simulink model "frequency_syn"  (R2016a)
settings: Solver=VariableStepAuto  StartTime=0.0  StopTime=10.0  RelTol=1e-3
undefined symbols (not defined in the file or in its folder): j
libraries: dspobslib x3, commchan3 x2, commdigbbndpm3 x1, commrandsrc2 x1, dspxfrm3 x1
settings Model: Creator=dell  LastModifiedBy=dell

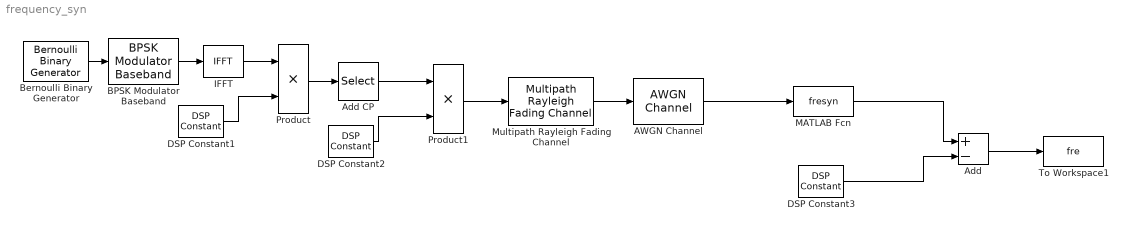
== system frequency_syn ==
  AWGN Channel : commchan3/AWGN Channel  InputProcessing=Inherited (this choice will be removed - see release notes)  seed=67  noiseMode="Signal to noise ratio  (SNR)"  EbNodB=ebn0  EsNodB=10  SNRdB=snr  bitsPerSym=1  Ps=1  Tsym=1/480000  variance=1
  Add : Sum  Inputs=+-
  Add CP : Selector  InputPortWidth=128  IndexOptions=Index vector (dialog)  Indices=[100:128 1:128]  OutputSizes=1
  BPSK Modulator Baseband : commdigbbndpm3/BPSK Modulator Baseband  Ph=0  outDtype=double  outWordLen=16  outUDDataType=sfix(16)  outFracLenMode=Best precision  outFracLen=15  outDataTypeStr=double  outLastDataTypeStr=double
  Bernoulli Binary Generator : commrandsrc2/Bernoulli Binary Generator  P=0.5  seed=565  Ts=1/480000  frameBased=on  sampPerFrame=128  orient=off  outDataType=double
  DSP Constant1 : dspobslib/DSP Constant  Value=sqrt(128)  SampleMode=Discrete  discreteOutput=Sample-based  continuousOutput=Sample-based  sampTime=inf  framePeriod=2  dataType=Inherit from 'Constant value'  isSigned=on  wordLen=16  udDataType=sfix(16)  fracBitsMode=Best precision  numFracBits=15  InterpretAs1D=-inf  Ts=-inf  FramebasedOutput=-inf
  DSP Constant2 : dspobslib/DSP Constant  Value=exp(j*2*pi*0.2*[1:157]'/128)  SampleMode=Discrete  discreteOutput=Sample-based  continuousOutput=Sample-based  sampTime=inf  framePeriod=2  dataType=Inherit from 'Constant value'  isSigned=on  wordLen=16  udDataType=sfix(16)  fracBitsMode=Best precision  numFracBits=15  InterpretAs1D=-inf  Ts=-inf  FramebasedOutput=-inf
  DSP Constant3 : dspobslib/DSP Constant  Value=0.2  SampleMode=Discrete  discreteOutput=Sample-based  continuousOutput=Sample-based  sampTime=inf  framePeriod=2  dataType=Inherit from 'Constant value'  isSigned=on  wordLen=16  udDataType=sfix(16)  fracBitsMode=Best precision  numFracBits=15  InterpretAs1D=-inf  Ts=-inf  FramebasedOutput=-inf
  IFFT : dspxfrm3/IFFT  FFTImplementation=Auto  CompMethod=Table lookup  TableOpt=HYBRID  TableOptActive=Speed  BitRevOrder=off  cs_in=off  Normalize=on  InheritFFTLength=on  FFTLength=64  WrapInput=on  mode=Complex  outSamplingMode=Frame based  roundingMode=Floor  overflowMode=off  firstCoeffDataTypeStr=Inherit: Same word length as input  firstCoeffLastDataTypeStr=Inherit: Same word length as input  outputMin=[]  outputMax=[]
  MATLAB Fcn : MATLABFcn  MATLABFcn=fresyn  Output1D=off
  Multipath Rayleigh Fading Channel : commchan3/Multipath Rayleigh Fading Channel  maxDopplerShift=40  spectrumType=Jakes  sigmaGaussian=1/sqrt(2)  coeffRounded=[1 -1.72 0.785]  freqMinMaxRJakes=[0 1]  freqMinMaxAJakes=[0 1]  sigmaGaussian1=1/sqrt(2)  sigmaGaussian2=1/sqrt(2)  centerFreqGaussian1=0.0  centerFreqGaussian2=0.0  gainGaussian1=0.5  gainGaussian2=0.5  coeffBell=9  dopplerSpectrum=doppler.jakes  pathDelays=[0 1e-6 2e-6]  avgPathGaindB=[0 -3 -9]  normalizePathGains=on  seed=73  enableProbe=0  openVisAtStart=off  outPathGains=off  outDelay=off
  Product : Product  RndMeth=Zero
  Product1 : Product  RndMeth=Zero
  To Workspace1 : ToWorkspace  VariableName=fre  SampleTime=-1
      settings: Save2DSignal=2-D array (concatenate along first dimension)
  wires:
  IFFT/1 -> Product/1
  DSP Constant1/1 -> Product/2
  Product/1 -> Add CP/1
  AWGN Channel/1 -> MATLAB Fcn/1
  Multipath Rayleigh Fading Channel/1 -> AWGN Channel/1
  Add CP/1 -> Product1/1
  DSP Constant2/1 -> Product1/2
  Product1/1 -> Multipath Rayleigh Fading Channel/1
  MATLAB Fcn/1 -> Add/1
  DSP Constant3/1 -> Add/2
  Add/1 -> To Workspace1/1
  Bernoulli Binary Generator/1 -> BPSK Modulator Baseband/1
  BPSK Modulator Baseband/1 -> IFFT/1
